simulink model "localDP_bs_env"  (R2020a)
settings: Solver=ode4  StartTime=0.0  StopTime=2000.0  FixedStep=1  RelTol=1e-3
InitFcn:
  | initial_data
values from neighbouring files (symbols this model uses):
  D1 = [MM1(1,1)/100, 0, 0; 0, MM1(2,2)/40, 0; 0, 0, MM1(3,3)/20]    [main.m]
  M1 = diag([6.25e5, 6.25e5, 6.25e5*7.5^2])    [main.m]
  Ma1 = [7.58e4, 0, 0; 0, 3.69e5 -1.4e5; 0, -1.4e5, 8.77e6]    [main.m]
undefined symbols (not defined in the file or in its folder): magnitude
libraries: simulink x2
settings Model: Creator=jiang  LastModifiedBy=jiang

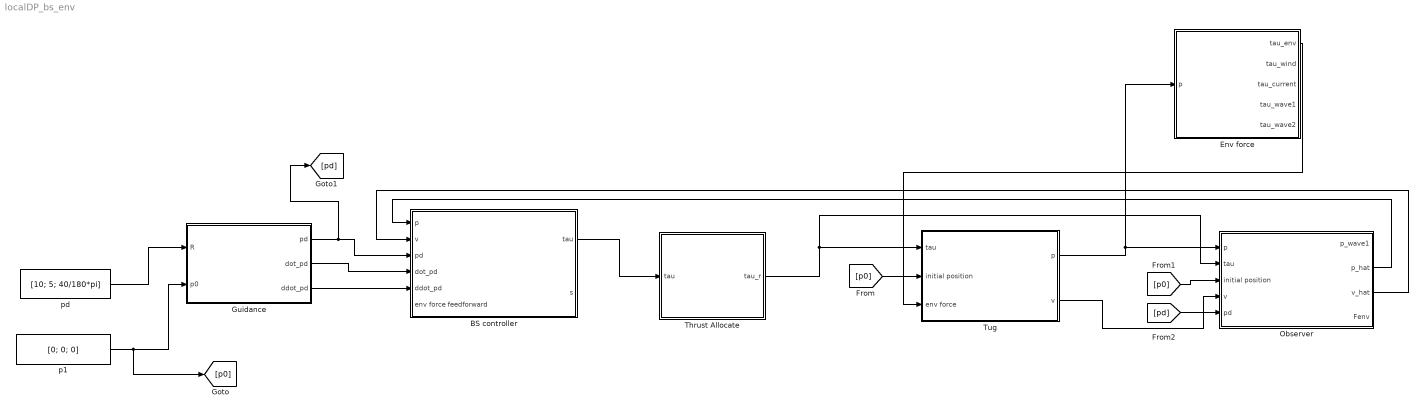
== system localDP_bs_env ==
  BS controller : Subsystem  mask{Kd=[2.5, 2.5, 2], Ki=[0.1, 0.1, 0.1], Gama=[0.7, 0.7, 0.7]}
      mask Display: disp("BS controller")
  Env force : Subsystem  mask{wind_speed=3, wind_angle=0, wind_ratio=0, current_speed=0.3, current_angle=0, current_ratio=0, wave_Hs=4.8, wave_Tp=13.4, wave_angle=0, wave1_ratio=1, wave2_ratio=1}
      mask prompts: wind_speed "wind speed"; wind_angle "wind angle"; wind_ratio "wind ratio"; current_speed "current speed"; current_angle "current angle"; current_ratio "current ratio"; wave_Hs "wave Hs"; wave_Tp "wave Tp"; wave_angle "wave angle"; wave1_ratio "wave1 ratio"; wave2_ratio "wave2 ratio"
      mask DialogControl ParameterGroupVar Prompt: wind parameters
      mask DialogControl Container5 Prompt: current parameters
      mask DialogControl wave Prompt: wave parameters
  Guidance : Subsystem  mask{T=[100, 100, 100]}
      mask prompts: T "时间常数"
  Observer : Subsystem  mask(wave spectrum damping ratio){lambda=[0.1 0.1 0.1], w_o=[0.469 0.469 0.469], K3=diag([1.4e4, 1.6e4, 2.5e6])*0.1, K4=diag([1.4e4, 1.6e4, 2.5e6]), w_c=0.6, T=diag([10 10 10])*100, Tp=13.4, wc_ratio=1.2}
      mask prompts: lambda "Relative damping ratio of wave spectrum: lambda"; w_o "Peak frequency of response spectrum: w_o (rad/s)"; K3 "Bias observer gain: K3"; K4 "Bias observer gain: K4"; w_c "Filter cut-off frequency: w_c (rad/s)"; T "Bias time constant: T (s)"; Tp "波浪谱峰周期"; wc_ratio "截至频率倍数（1.1~1.2）"
      mask init:
      | wo = [1, 1, 1] * 2 * pi / Tp;
      | wc = wo(1) * wc_ratio;
      | Zeta = 1;
      | Aw = blkdiag([0 1;-wo(1)^2 -2*lambda(1)*wo(1)],...
      |              [0 1;-wo(2)^2 -2*lambda(2)*wo(2)],...
      |              [0 1;-wo(3)^2 -2*lambda(3)*wo(3)]);
      | K1 = zeros(6,3);
      | for i =1:3
      |     K1(2*i-1,i) = -2*(Zeta - lambda(i))*wc/wo(i);
      |     K1(2*i,i) = 2*wo(i)*(Zeta - lambda(i));
      | end
      | K2 = diag([wc,wc,wc]);
      | Cw = zeros(3,6);
      | Cw(1,2) = 1;Cw(2,4) = 1;Cw(3,6) = 1;
      mask Display: disp('nonlinear passive observer')
  Thrust Allocate : Subsystem  mask{f0=[100;100;100], a0=[-50;60;-100]}
  Tug : Subsystem  mask{wv=on}
      mask prompts: wv "Display animation of the vessel's motion"
  p1 : Constant  Value=[0; 0; 0]
  pd : Constant  Value=[10; 5; 40/180*pi]
  wires:
  Thrust Allocate/1(tau_r) -> Observer/2(tau), Tug/1(tau)
  BS controller/1(tau) -> Thrust Allocate/1(tau)
  Env force/1(tau_env) -> Tug/3(env force)
  Tug/2(v) -> Observer/4(v)
  Tug/1(p) -> Env force/1(p), Observer/1(p)
  Observer/2(p_hat) -> BS controller/1(p)
  Observer/3(v_hat) -> BS controller/2(v)
  p1/1 -> [p0], Guidance/2(p0)
  pd/1 -> Guidance/1(R)
  Guidance/2(dot_pd) -> BS controller/4(dot_pd)
  Guidance/1(pd) -> [pd], BS controller/3(pd)
  Guidance/3(ddot_pd) -> BS controller/5(ddot_pd)
  [p0] -> Tug/2(initial position)
  [p0] -> Observer/3(initial position)
  [pd] -> Observer/5(pd)

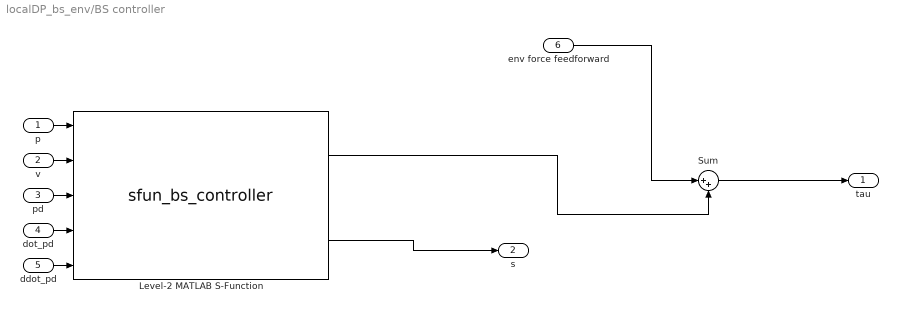
== system localDP_bs_env/BS controller ==
  p : Inport
  v : Inport  Port=2
  pd : Inport  Port=3
  dot_pd : Inport  Port=4
  ddot_pd : Inport  Port=5
  env force feedforward : Inport  Port=6
  Level-2 MATLAB S-Function : M-S-Function  FunctionName=sfun_bs_controller  Parameters=Kd, Ki, Gama
  Sum : Sum  Inputs=|++
  tau : Outport
  s : Outport  Port=2
  wires:
  Level-2 MATLAB S-Function/2 -> s/1
  v/1 -> Level-2 MATLAB S-Function/2
  p/1 -> Level-2 MATLAB S-Function/1
  pd/1 -> Level-2 MATLAB S-Function/3
  ddot_pd/1 -> Level-2 MATLAB S-Function/5
  dot_pd/1 -> Level-2 MATLAB S-Function/4
  Sum/1 -> tau/1
  Level-2 MATLAB S-Function/1 -> Sum/2
  env force feedforward/1 -> Sum/1

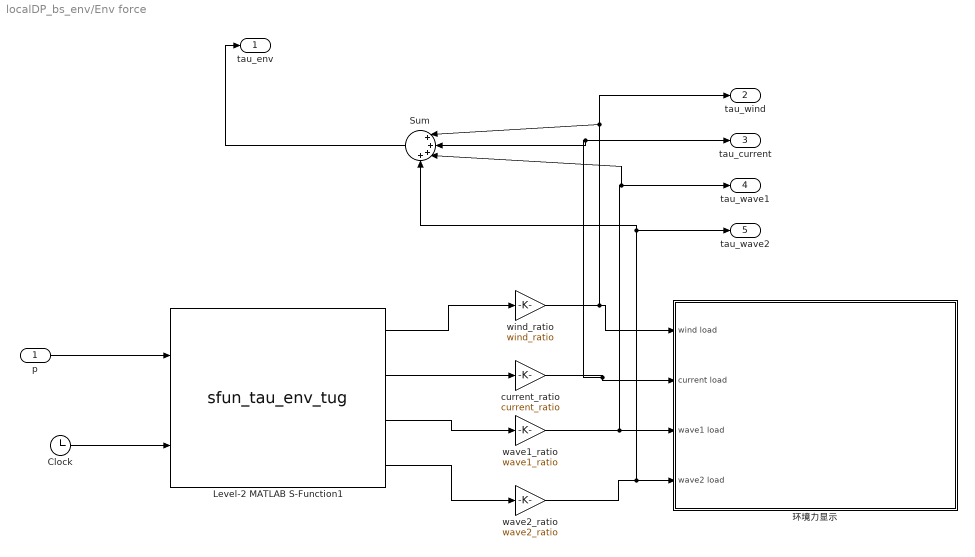
== system localDP_bs_env/Env force ==
  p : Inport
  Clock : Clock
  Level-2 MATLAB S-Function1 : M-S-Function  FunctionName=sfun_tau_env_tug  Parameters=wind_speed, wind_angle, current_speed, current_angle, wave_Hs, wave_Tp, wave_angle
  Sum : Sum  Inputs=|++++
  current_ratio : Gain  Gain=current_ratio
  wave1_ratio : Gain  Gain=wave1_ratio
  wave2_ratio : Gain  Gain=wave2_ratio
  wind_ratio : Gain  Gain=wind_ratio
  环境力显示 : Subsystem
  tau_env : Outport
  tau_wind : Outport  Port=2
  tau_current : Outport  Port=3
  tau_wave1 : Outport  Port=4
  tau_wave2 : Outport  Port=5
  wires:
  p/1 -> Level-2 MATLAB S-Function1/1
  Level-2 MATLAB S-Function1/1 -> wind_ratio/1
  Level-2 MATLAB S-Function1/2 -> current_ratio/1
  Level-2 MATLAB S-Function1/3 -> wave1_ratio/1
  Level-2 MATLAB S-Function1/4 -> wave2_ratio/1
  Clock/1 -> Level-2 MATLAB S-Function1/2
  wind_ratio/1 -> 环境力显示/1(wind load), tau_wind/1, Sum/1
  current_ratio/1 -> Sum/2, tau_current/1, 环境力显示/2(current load)
  wave1_ratio/1 -> Sum/3, tau_wave1/1, 环境力显示/3(wave1 load)
  wave2_ratio/1 -> Sum/4, tau_wave2/1, 环境力显示/4(wave2 load)
  Sum/1 -> tau_env/1

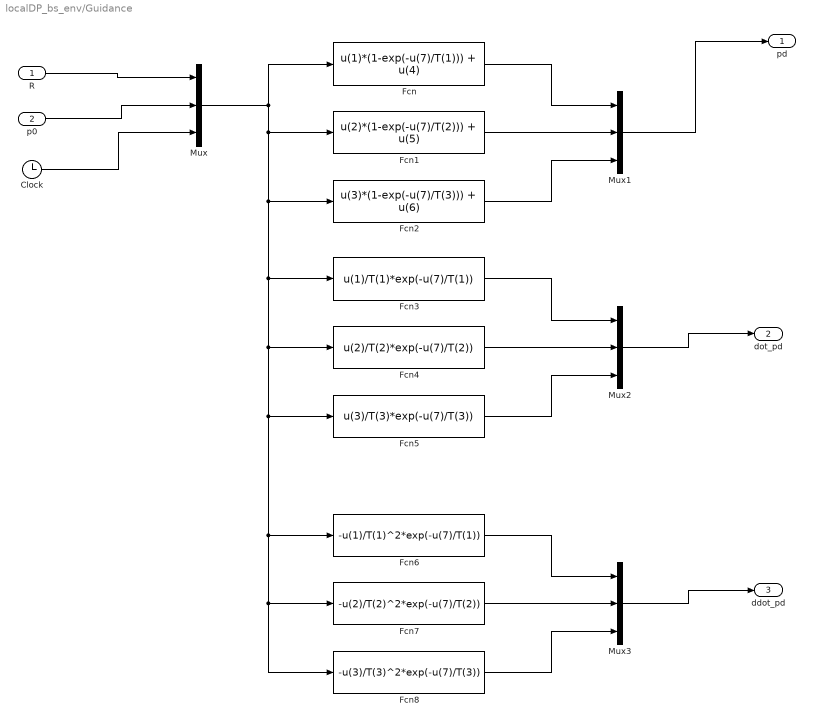
== system localDP_bs_env/Guidance ==
  R : Inport
  p0 : Inport  Port=2
  Clock : Clock
  Fcn : Fcn  Expr=u(1)*(1-exp(-u(7)/T(1))) + u(4)
  Fcn1 : Fcn  Expr=u(2)*(1-exp(-u(7)/T(2))) + u(5)
  Fcn2 : Fcn  Expr=u(3)*(1-exp(-u(7)/T(3))) + u(6)
  Fcn3 : Fcn  Expr=u(1)/T(1)*exp(-u(7)/T(1))
  Fcn4 : Fcn  Expr=u(2)/T(2)*exp(-u(7)/T(2))
  Fcn5 : Fcn  Expr=u(3)/T(3)*exp(-u(7)/T(3))
  Fcn6 : Fcn  Expr=-u(1)/T(1)^2*exp(-u(7)/T(1))
  Fcn7 : Fcn  Expr=-u(2)/T(2)^2*exp(-u(7)/T(2))
  Fcn8 : Fcn  Expr=-u(3)/T(3)^2*exp(-u(7)/T(3))
  Mux{,1..3} (4 alike) : Mux  Inputs=3
  pd : Outport
  dot_pd : Outport  Port=2
  ddot_pd : Outport  Port=3
  wires:
  Clock/1 -> Mux/3
  p0/1 -> Mux/2
  R/1 -> Mux/1
  Fcn/1 -> Mux1/1
  Fcn1/1 -> Mux1/2
  Fcn2/1 -> Mux1/3
  Mux1/1 -> pd/1
  Fcn5/1 -> Mux2/3
  Fcn4/1 -> Mux2/2
  Fcn3/1 -> Mux2/1
  Mux2/1 -> dot_pd/1
  Fcn7/1 -> Mux3/2
  Fcn6/1 -> Mux3/1
  Mux3/1 -> ddot_pd/1
  Mux/1 -> Fcn8/1, Fcn7/1, Fcn6/1, Fcn5/1, Fcn4/1, Fcn3/1, Fcn2/1, Fcn1/1, Fcn/1
  Fcn8/1 -> Mux3/3

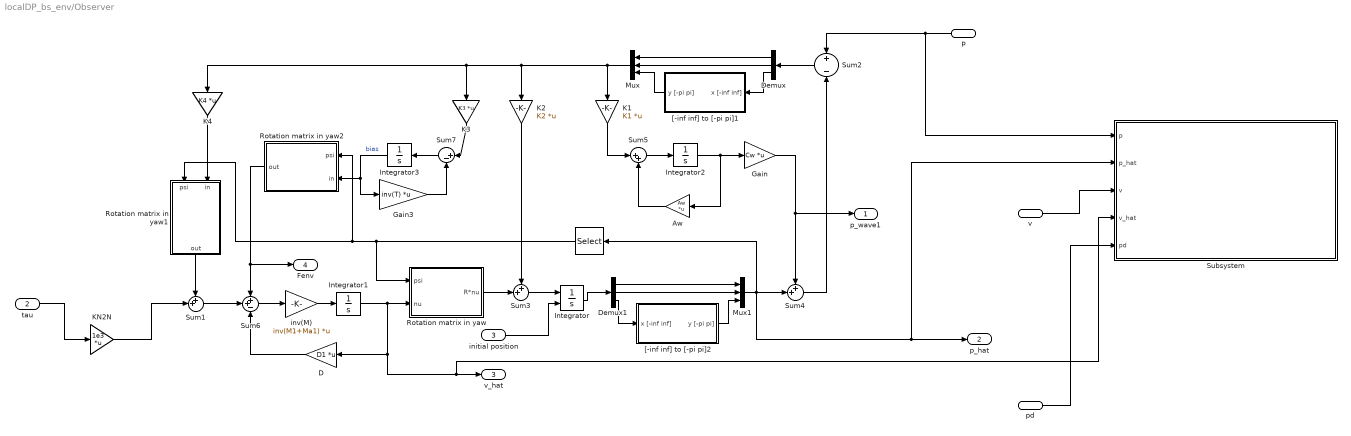
== system localDP_bs_env/Observer ==
  p : Inport
  tau : Inport  Port=2
  initial position : Inport  Port=3
  v : Inport  Port=4
  pd : Inport  Port=5
  " " : Selector  InputPortWidth=3  IndexOptions=Index vector (dialog)  Indices=[3]  OutputSizes=1
  Aw : Gain  Gain=Aw  Multiplication=Matrix(K*u)  SaturateOnIntegerOverflow=on  OutDataTypeStr=Inherit: Same as input  ParamDataTypeStr=Inherit: Same as input
  D : Gain  Gain=D1  Multiplication=Matrix(K*u)  SaturateOnIntegerOverflow=on  OutDataTypeStr=Inherit: Same as input  ParamDataTypeStr=Inherit: Same as input
  Demux : Demux  Outputs=3
  Demux1 : Demux  Outputs=3
  Gain : Gain  Gain=Cw  Multiplication=Matrix(K*u)
  Gain3 : Gain  Gain=inv(T)  Multiplication=Matrix(K*u)  SaturateOnIntegerOverflow=on  OutDataTypeStr=Inherit: Same as input  ParamDataTypeStr=Inherit: Same as input
  Integrator : Integrator  InitialConditionSource=external
  Integrator1 : Integrator
  Integrator2 : Integrator
  Integrator3 : Integrator
  K1 : Gain  Gain=K1  Multiplication=Matrix(K*u)  SaturateOnIntegerOverflow=on  OutDataTypeStr=Inherit: Same as input  ParamDataTypeStr=Inherit: Same as input
  K2 : Gain  Gain=K2  Multiplication=Matrix(K*u)  SaturateOnIntegerOverflow=on  OutDataTypeStr=Inherit: Same as input  ParamDataTypeStr=Inherit: Same as input
  K3 : Gain  Gain=K3  Multiplication=Matrix(K*u)  SaturateOnIntegerOverflow=on  OutDataTypeStr=Inherit: Same as input  ParamDataTypeStr=Inherit: Same as input
  K4 : Gain  Gain=K4  Multiplication=Matrix(K*u)  SaturateOnIntegerOverflow=on  OutDataTypeStr=Inherit: Same as input  ParamDataTypeStr=Inherit: Same as input
  KN2N : Gain  Gain=1e3  Multiplication=Matrix(K*u)  SaturateOnIntegerOverflow=on  OutDataTypeStr=Inherit: Same as input  ParamDataTypeStr=Inherit: Same as input
  Mux : Mux  Inputs=3
  Mux1 : Mux  Inputs=3
  Rotation matrix in yaw : Subsystem
  Rotation matrix in yaw1 : Subsystem
  Rotation matrix in yaw2 : Subsystem
  Subsystem : Subsystem
  Sum1 : Sum  Inputs=++|  InputSameDT=on  SaturateOnIntegerOverflow=on  OutDataTypeStr=Inherit: Same as first input
  Sum2 : Sum  Inputs=+|-  InputSameDT=on  SaturateOnIntegerOverflow=on  OutDataTypeStr=Inherit: Same as first input
  Sum3 : Sum  Inputs=++|  InputSameDT=on  SaturateOnIntegerOverflow=on  OutDataTypeStr=Inherit: Same as first input
  Sum4 : Sum  Inputs=++|  InputSameDT=on  SaturateOnIntegerOverflow=on  OutDataTypeStr=Inherit: Same as first input
  Sum5 : Sum  Inputs=|++  InputSameDT=on  SaturateOnIntegerOverflow=on  OutDataTypeStr=Inherit: Same as first input
  Sum6 : Sum  Inputs=++-  InputSameDT=on  SaturateOnIntegerOverflow=on  OutDataTypeStr=Inherit: Same as first input
  Sum7 : Sum  Inputs=|+-  InputSameDT=on  SaturateOnIntegerOverflow=on  OutDataTypeStr=Inherit: Same as first input
  "[-inf inf] to [-pi pi]1" : Subsystem  mask([-inf inf] to [-pi pi]){}
      mask help: Converts an angle in rad to (-pi pi)
  "[-inf inf] to [-pi pi]2" : Subsystem
  inv(M) : Gain  Gain=inv(M1+Ma1)  Multiplication=Matrix(K*u)  SaturateOnIntegerOverflow=on  OutDataTypeStr=Inherit: Same as input  ParamDataTypeStr=Inherit: Same as input
  p_wave1 : Outport
  p_hat : Outport  Port=2
  v_hat : Outport  Port=3
  Fenv : Outport  Port=4
  wires:
  tau/1 -> KN2N/1
  p/1 -> Subsystem/1(p), Sum2/1
  Gain3/1 -> Sum7/2
  Sum7/1 -> Integrator3/1
  Integrator3/1 -> Gain3/1, Rotation matrix in yaw2/2(in)  "bias"
  Sum4/1 -> Sum2/2
  Integrator/1 -> Demux1/1
  Sum3/1 -> Integrator/1
  Sum2/1 -> Demux/1
  Demux/3 -> "[-inf inf] to [-pi pi]1"/1(x [-inf inf])
  "[-inf inf] to [-pi pi]1"/1(y [-pi pi]) -> Mux/3
  Demux/1 -> Mux/1
  Demux/2 -> Mux/2
  Mux/1 -> K1/1, K2/1, K4/1, K3/1
  Demux1/1 -> Mux1/1
  Demux1/2 -> Mux1/2
  "[-inf inf] to [-pi pi]2"/1(y [-pi pi]) -> Mux1/3
  Demux1/3 -> "[-inf inf] to [-pi pi]2"/1(x [-inf inf])
  Mux1/1 -> Subsystem/2(p_hat), p_hat/1, Sum4/2, " "/1
  Sum5/1 -> Integrator2/1
  K1/1 -> Sum5/1
  Integrator2/1 -> Gain/1, Aw/1
  Aw/1 -> Sum5/2
  K2/1 -> Sum3/1
  Rotation matrix in yaw/1(R*nu) -> Sum3/2
  K3/1 -> Sum7/1
  inv(M)/1 -> Integrator1/1
  Sum6/1 -> inv(M)/1
  Integrator1/1 -> Rotation matrix in yaw/2(nu), D/1, Subsystem/4(v_hat), v_hat/1
  " "/1 -> Rotation matrix in yaw/1(psi), Rotation matrix in yaw1/1(psi), Rotation matrix in yaw2/1(psi)
  Sum1/1 -> Sum6/2
  D/1 -> Sum6/3
  K4/1 -> Rotation matrix in yaw1/2(in)
  Rotation matrix in yaw1/1(out) -> Sum1/1
  Rotation matrix in yaw2/1(out) -> Sum6/1, Fenv/1
  initial position/1 -> Integrator/2
  Gain/1 -> Sum4/1, p_wave1/1
  v/1 -> Subsystem/3(v)
  KN2N/1 -> Sum1/2
  pd/1 -> Subsystem/5(pd)

== system localDP_bs_env/Thrust Allocate ==
  tau : Inport
  Comparison between thrusts : Subsystem
  Level-2 MATLAB S-Function : M-S-Function  FunctionName=sfun_Thrust_Allocate  Parameters=f0, a0
  a : Scope
  f : Scope
  tau1 : Scope  NumInputPorts=3
  tau_r : Outport
  wires:
  tau/1 -> Comparison between thrusts/1(commanded thrust), Level-2 MATLAB S-Function/1
  Level-2 MATLAB S-Function/5 -> Comparison between thrusts/2(real thrust), tau_r/1
  Level-2 MATLAB S-Function/1 -> f/1
  Level-2 MATLAB S-Function/3 -> a/1
  Comparison between thrusts/1(surge direction) -> tau1/1
  Comparison between thrusts/2(sway direction) -> tau1/2
  Comparison between thrusts/3(yaw direction) -> tau1/3

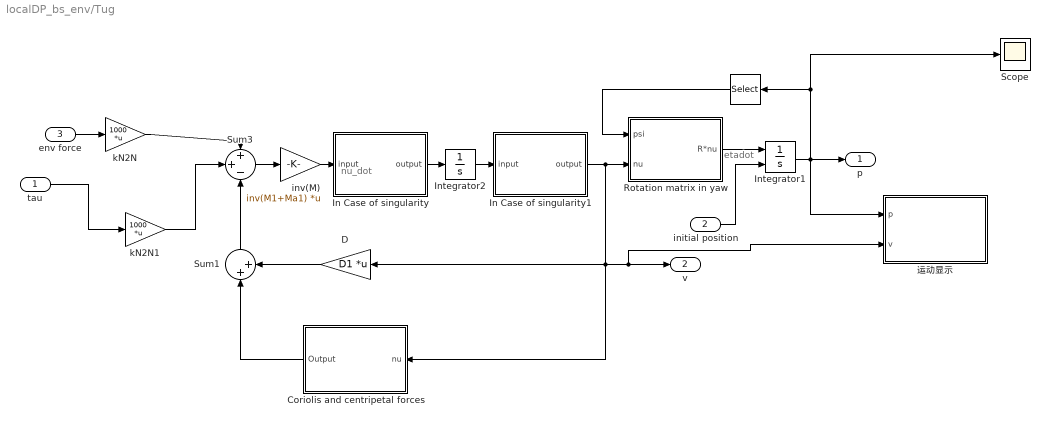
== system localDP_bs_env/Tug ==
  note: nu_dot
  note: etadot
  tau : Inport
  initial position : Inport  Port=2
  env force : Inport  Port=3
  " " : Selector  InputPortWidth=3  IndexOptions=Index vector (dialog)  Indices=[3]  OutputSizes=1
  Coriolis and centripetal forces : Subsystem
  D : Gain  Gain=D1  Multiplication=Matrix(K*u)  SaturateOnIntegerOverflow=on  OutDataTypeStr=Inherit: Same as input  ParamDataTypeStr=Inherit: Same as input
  In Case of singularity : Subsystem
  In Case of singularity1 : Subsystem
  Integrator1 : Integrator  InitialConditionSource=external  InitialCondition=1.05
  Integrator2 : Integrator
  Rotation matrix in yaw : Subsystem
  Scope : Scope
  Sum1 : Sum  Inputs=|++  InputSameDT=on  SaturateOnIntegerOverflow=on  OutDataTypeStr=Inherit: Same as first input
  Sum3 : Sum  Inputs=++-  InputSameDT=on  SaturateOnIntegerOverflow=on  OutDataTypeStr=Inherit: Same as first input
  inv(M) : Gain  Gain=inv(M1+Ma1)  Multiplication=Matrix(K*u)  SaturateOnIntegerOverflow=on  OutDataTypeStr=Inherit: Same as input  ParamDataTypeStr=Inherit: Same as input
  kN2N : Gain  Gain=1000  Multiplication=Matrix(K*u)  SaturateOnIntegerOverflow=on  OutDataTypeStr=Inherit: Same as input  ParamDataTypeStr=Inherit: Same as input
  kN2N1 : Gain  Gain=1000  Multiplication=Matrix(K*u)  SaturateOnIntegerOverflow=on  OutDataTypeStr=Inherit: Same as input  ParamDataTypeStr=Inherit: Same as input
  运动显示 : Subsystem
  p : Outport
  v : Outport  Port=2
  wires:
  Sum3/1 -> inv(M)/1
  inv(M)/1 -> In Case of singularity/1(input)
  Rotation matrix in yaw/1(R*nu) -> Integrator1/1
  Integrator1/1 -> 运动显示/1(p), p/1, Scope/1, " "/1
  " "/1 -> Rotation matrix in yaw/1(psi)
  tau/1 -> kN2N1/1
  initial position/1 -> Integrator1/2
  Sum1/1 -> Sum3/3
  env force/1 -> kN2N/1
  Integrator2/1 -> In Case of singularity1/1(input)
  In Case of singularity/1(output) -> Integrator2/1
  In Case of singularity1/1(output) -> Rotation matrix in yaw/2(nu), D/1, Coriolis and centripetal forces/1(nu), 运动显示/2(v), v/1
  D/1 -> Sum1/2
  Coriolis and centripetal forces/1(Output) -> Sum1/1
  kN2N/1 -> Sum3/1
  kN2N1/1 -> Sum3/2

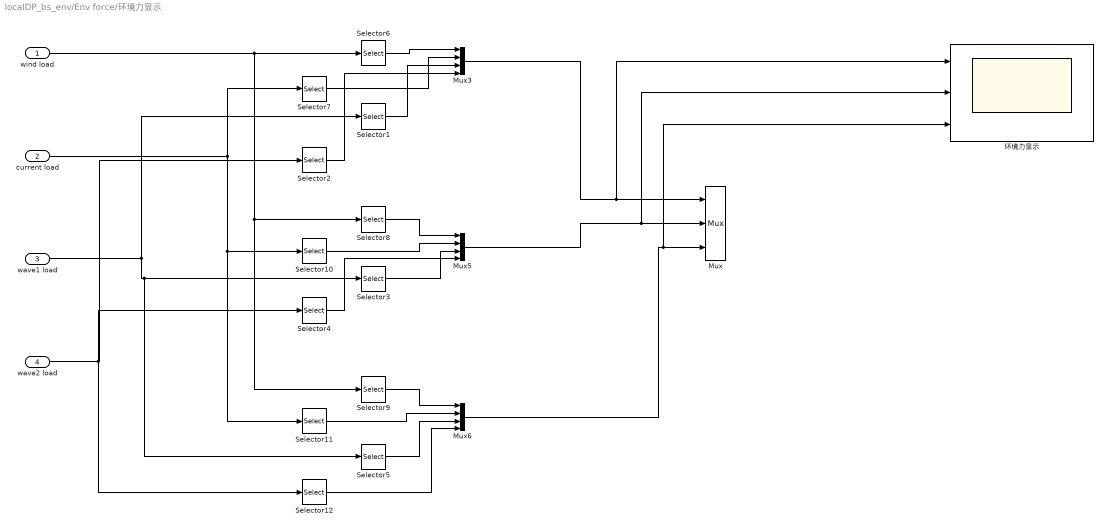
== system localDP_bs_env/Env force/环境力显示 ==
  wind load : Inport
  current load : Inport  Port=2
  wave1 load : Inport  Port=3
  wave2 load : Inport  Port=4
  Mux : Mux  Inputs=3
  Mux3 : Mux
  Mux5 : Mux
  Mux6 : Mux
  Selector{1..2,6..7} (4 alike) : Selector  InputPortWidth=3  IndexOptions=Index vector (dialog)  Indices=[1]  OutputSizes=1
  Selector{3..4,8,10} (4 alike) : Selector  InputPortWidth=3  IndexOptions=Index vector (dialog)  Indices=[2]  OutputSizes=1
  Selector{5,9,11..12} (4 alike) : Selector  InputPortWidth=3  IndexOptions=Index vector (dialog)  Indices=[3]  OutputSizes=1
  环境力显示 : Scope  NumInputPorts=3
  wires:
  Selector8/1 -> Mux5/1
  Mux3/1 -> 环境力显示/1, Mux/1
  Selector10/1 -> Mux5/2
  wind load/1 -> Selector9/1, Selector8/1, Selector6/1
  Selector7/1 -> Mux3/2
  Selector6/1 -> Mux3/1
  Selector9/1 -> Mux6/1
  Selector11/1 -> Mux6/2
  current load/1 -> Selector11/1, Selector10/1, Selector7/1
  Mux5/1 -> 环境力显示/2, Mux/2
  Mux6/1 -> 环境力显示/3, Mux/3
  wave1 load/1 -> Selector1/1, Selector5/1, Selector3/1
  Selector1/1 -> Mux3/3
  Selector2/1 -> Mux3/4
  Selector3/1 -> Mux5/3
  wave2 load/1 -> Selector12/1, Selector4/1, Selector2/1
  Selector4/1 -> Mux5/4
  Selector5/1 -> Mux6/3
  Selector12/1 -> Mux6/4

== system localDP_bs_env/Observer/Rotation matrix in yaw ==
  psi : Inport
  nu : Inport  Port=2
  Fcn : Fcn  Expr=cos(u(1))*u(2)-sin(u(1))*u(3)
  Fcn1 : Fcn  Expr=sin(u(1))*u(2)+cos(u(1))*u(3)
  Fcn2 : Fcn  Expr=u(4)
  Mux : Mux  Inputs=2
  Mux1 : Mux  Inputs=3
  R*nu : Outport
  wires:
  Mux1/1 -> R*nu/1  "eta_dot"
  Mux/1 -> Fcn/1, Fcn1/1, Fcn2/1
  psi/1 -> Mux/1
  nu/1 -> Mux/2
  Fcn1/1 -> Mux1/2  "y_dot"
  Fcn/1 -> Mux1/1  "x_dot"
  Fcn2/1 -> Mux1/3  "psi_dot"

== system localDP_bs_env/Observer/Rotation matrix in yaw1 ==
  psi : Inport
  in : Inport  Port=2
  Fcn : Fcn  Expr=cos(u(1))*u(2)+sin(u(1))*u(3)
  Fcn1 : Fcn  Expr=-sin(u(1))*u(2)+cos(u(1))*u(3)
  Fcn2 : Fcn  Expr=u(4)
  Mux : Mux  Inputs=2
  Mux1 : Mux  Inputs=3
  out : Outport
  wires:
  Fcn2/1 -> Mux1/3
  Fcn/1 -> Mux1/1
  Fcn1/1 -> Mux1/2
  in/1 -> Mux/2
  psi/1 -> Mux/1
  Mux/1 -> Fcn2/1, Fcn1/1, Fcn/1
  Mux1/1 -> out/1

== system localDP_bs_env/Observer/Rotation matrix in yaw2 ==
  psi : Inport
  in : Inport  Port=2
  Fcn : Fcn  Expr=cos(u(1))*u(2)+sin(u(1))*u(3)
  Fcn1 : Fcn  Expr=-sin(u(1))*u(2)+cos(u(1))*u(3)
  Fcn2 : Fcn  Expr=u(4)
  Mux : Mux  Inputs=2
  Mux1 : Mux  Inputs=3
  out : Outport
  wires:
  Mux1/1 -> out/1
  Mux/1 -> Fcn/1, Fcn1/1, Fcn2/1
  psi/1 -> Mux/1
  in/1 -> Mux/2
  Fcn1/1 -> Mux1/2
  Fcn/1 -> Mux1/1
  Fcn2/1 -> Mux1/3

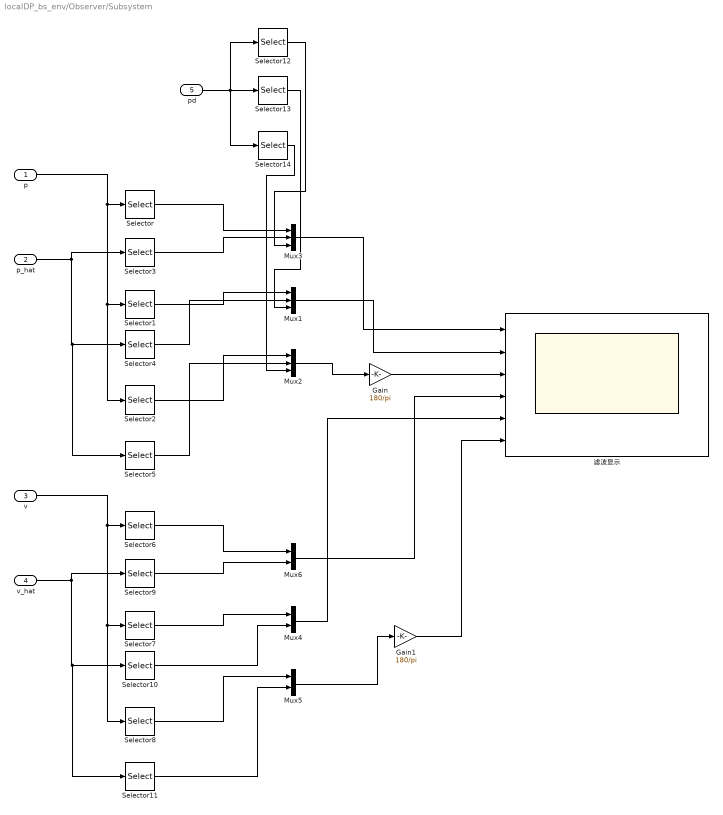
== system localDP_bs_env/Observer/Subsystem ==
  p : Inport
  p_hat : Inport  Port=2
  v : Inport  Port=3
  v_hat : Inport  Port=4
  pd : Inport  Port=5
  Gain : Gain  Gain=180/pi
  Gain1 : Gain  Gain=180/pi
  Mux1 : Mux  Inputs=3
  Mux2 : Mux  Inputs=3
  Mux3 : Mux  Inputs=3
  Mux4 : Mux  Inputs=2
  Mux5 : Mux  Inputs=2
  Mux6 : Mux  Inputs=2
  Selector{,3,6,9,12} (5 alike) : Selector  InputPortWidth=3  IndexOptions=Index vector (dialog)  Indices=[1 ]  OutputSizes=1
  Selector{1,4,7,10,13} (5 alike) : Selector  InputPortWidth=3  IndexOptions=Index vector (dialog)  Indices=[2 ]  OutputSizes=1
  Selector{2,5,8,11,14} (5 alike) : Selector  InputPortWidth=3  IndexOptions=Index vector (dialog)  Indices=[3 ]  OutputSizes=1
  滤波显示 : Scope  NumInputPorts=6
  wires:
  p/1 -> Selector2/1, Selector1/1, Selector/1
  Selector/1 -> Mux3/1
  p_hat/1 -> Selector5/1, Selector4/1, Selector3/1
  Selector3/1 -> Mux3/2
  Mux3/1 -> 滤波显示/1
  Mux1/1 -> 滤波显示/2
  Mux2/1 -> Gain/1
  Mux5/1 -> Gain1/1
  v/1 -> Selector8/1, Selector7/1, Selector6/1
  v_hat/1 -> Selector11/1, Selector10/1, Selector9/1
  Mux6/1 -> 滤波显示/4
  Mux4/1 -> 滤波显示/5
  Selector1/1 -> Mux1/1
  Selector4/1 -> Mux1/2
  Selector2/1 -> Mux2/1
  Selector5/1 -> Mux2/2
  Selector6/1 -> Mux6/1
  Selector9/1 -> Mux6/2
  Selector7/1 -> Mux4/1
  Selector10/1 -> Mux4/2
  Selector8/1 -> Mux5/1
  Selector11/1 -> Mux5/2
  Gain/1 -> 滤波显示/3
  Gain1/1 -> 滤波显示/6
  pd/1 -> Selector14/1, Selector13/1, Selector12/1
  Selector12/1 -> Mux3/3
  Selector13/1 -> Mux1/3
  Selector14/1 -> Mux2/3

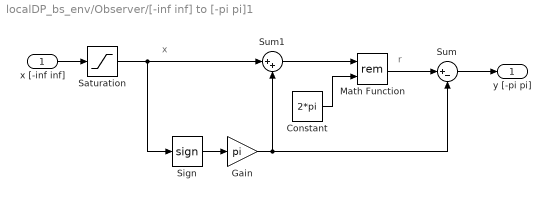
== system localDP_bs_env/Observer/[-inf inf] to [-pi pi]1 ==
  note: x
  note: r
  x [-inf inf] : Inport
  Constant : Constant  Value=2*pi
  Gain : Gain  Gain=pi  SaturateOnIntegerOverflow=on  OutDataTypeStr=Inherit: Same as input  ParamDataTypeStr=Inherit: Same as input
  Math Function : Math  Operator=rem  SignedPower=on  SaturateOnIntegerOverflow=on
  Saturation : Saturate  UpperLimit=1e10  LowerLimit=-1e10
  Sign : Signum
  Sum : Sum  Inputs=|+-  SaturateOnIntegerOverflow=on
  Sum1 : Sum  Inputs=|++  SaturateOnIntegerOverflow=on
  y [-pi pi] : Outport
  wires:
  x [-inf inf]/1 -> Saturation/1
  Sign/1 -> Gain/1
  Gain/1 -> Sum/2, Sum1/2
  Sum1/1 -> Math Function/1
  Constant/1 -> Math Function/2
  Math Function/1 -> Sum/1
  Sum/1 -> y [-pi pi]/1
  Saturation/1 -> Sum1/1, Sign/1

== system localDP_bs_env/Observer/[-inf inf] to [-pi pi]2 ==
  note: r
  note: x
  x [-inf inf] : Inport
  Constant : Constant  Value=2*pi
  Gain : Gain  Gain=pi  SaturateOnIntegerOverflow=on  OutDataTypeStr=Inherit: Same as input  ParamDataTypeStr=Inherit: Same as input
  Math Function : Math  Operator=rem  SignedPower=on  SaturateOnIntegerOverflow=on
  Saturation : Saturate  UpperLimit=1e10  LowerLimit=-1e10
  Sign : Signum
  Sum : Sum  Inputs=|+-  SaturateOnIntegerOverflow=on
  Sum1 : Sum  Inputs=|++  SaturateOnIntegerOverflow=on
  y [-pi pi] : Outport
  wires:
  Saturation/1 -> Sign/1, Sum1/1
  Sum/1 -> y [-pi pi]/1
  Math Function/1 -> Sum/1
  Constant/1 -> Math Function/2
  Sum1/1 -> Math Function/1
  Gain/1 -> Sum1/2, Sum/2
  Sign/1 -> Gain/1
  x [-inf inf]/1 -> Saturation/1

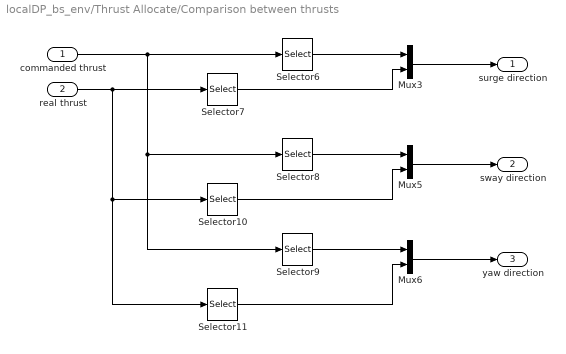
== system localDP_bs_env/Thrust Allocate/Comparison between thrusts ==
  commanded thrust : Inport
  real thrust : Inport  Port=2
  Mux3 : Mux  Inputs=2
  Mux5 : Mux  Inputs=2
  Mux6 : Mux  Inputs=2
  Selector10 : Selector  InputPortWidth=3  IndexOptions=Index vector (dialog)  Indices=[2]  OutputSizes=1
  Selector11 : Selector  InputPortWidth=3  IndexOptions=Index vector (dialog)  Indices=[3]  OutputSizes=1
  Selector6 : Selector  InputPortWidth=3  IndexOptions=Index vector (dialog)  Indices=[1]  OutputSizes=1
  Selector7 : Selector  InputPortWidth=3  IndexOptions=Index vector (dialog)  Indices=[1]  OutputSizes=1
  Selector8 : Selector  InputPortWidth=3  IndexOptions=Index vector (dialog)  Indices=[2]  OutputSizes=1
  Selector9 : Selector  InputPortWidth=3  IndexOptions=Index vector (dialog)  Indices=[3]  OutputSizes=1
  surge direction : Outport
  sway direction : Outport  Port=2
  yaw direction : Outport  Port=3
  wires:
  Selector9/1 -> Mux6/1
  Selector11/1 -> Mux6/2
  Selector10/1 -> Mux5/2
  Selector8/1 -> Mux5/1
  Selector7/1 -> Mux3/2
  Selector6/1 -> Mux3/1
  Mux3/1 -> surge direction/1
  Mux5/1 -> sway direction/1
  Mux6/1 -> yaw direction/1
  commanded thrust/1 -> Selector6/1, Selector8/1, Selector9/1
  real thrust/1 -> Selector7/1, Selector10/1, Selector11/1

== system localDP_bs_env/Tug/Coriolis and centripetal forces ==
  nu : Inport
  Mux : Mux  Inputs=3
  Selector1 : Selector  InputPortWidth=3  IndexOptions=Index vector (dialog)  Indices=[1 ]  OutputSizes=1
  Selector2 : Selector  InputPortWidth=3  IndexOptions=Index vector (dialog)  Indices=[2]  OutputSizes=1
  Selector3 : Selector  InputPortWidth=3  IndexOptions=Index vector (dialog)  Indices=[3]  OutputSizes=1
  Subsystem : Subsystem
  Subsystem1 : Subsystem
  Subsystem2 : Subsystem
  Output : Outport
  wires:
  nu/1 -> Selector1/1, Selector2/1, Selector3/1
  Selector2/1 -> Subsystem/1(v), Subsystem2/2(v)  "v"
  Selector3/1 -> Subsystem/2(r), Subsystem1/2(r), Subsystem2/3(r)  "r"
  Selector1/1 -> Subsystem1/1(u), Subsystem2/1(u)  "u"
  Subsystem/1(x direction) -> Mux/1
  Subsystem1/1(y direction) -> Mux/2
  Subsystem2/1(yaw direction) -> Mux/3
  Mux/1 -> Output/1

== system localDP_bs_env/Tug/In Case of singularity ==
  input : Inport
  Compare To Constant : simulink/Logic and Bit Operations/Compare To Constant  relop=>=  const=1e8  OutDataTypeStr=boolean
  Stop Simulation : Stop
  output : Outport
  wires:
  input/1 -> output/1, Compare To Constant/1
  Compare To Constant/1 -> Stop Simulation/1

== system localDP_bs_env/Tug/In Case of singularity1 ==
  input : Inport
  Compare To Constant : simulink/Logic and Bit Operations/Compare To Constant  relop=>=  const=1e10  OutDataTypeStr=boolean
  Stop Simulation : Stop
  output : Outport
  wires:
  input/1 -> output/1, Compare To Constant/1
  Compare To Constant/1 -> Stop Simulation/1

== system localDP_bs_env/Tug/Rotation matrix in yaw ==
  psi : Inport
  nu : Inport  Port=2
  Fcn : Fcn  Expr=cos(u(1))*u(2)-sin(u(1))*u(3)
  Fcn1 : Fcn  Expr=sin(u(1))*u(2)+cos(u(1))*u(3)
  Fcn2 : Fcn  Expr=u(4)
  Mux : Mux  Inputs=2
  Mux1 : Mux  Inputs=3
  R*nu : Outport
  wires:
  Mux1/1 -> R*nu/1  "eta_dot"
  Mux/1 -> Fcn/1, Fcn1/1, Fcn2/1
  psi/1 -> Mux/1
  nu/1 -> Mux/2
  Fcn1/1 -> Mux1/2  "y_dot"
  Fcn/1 -> Mux1/1  "x_dot"
  Fcn2/1 -> Mux1/3  "psi_dot"

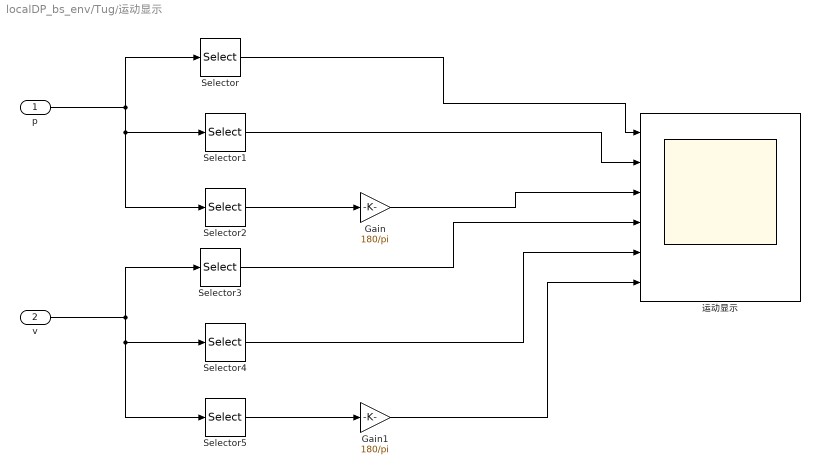
== system localDP_bs_env/Tug/运动显示 ==
  p : Inport
  v : Inport  Port=2
  Gain : Gain  Gain=180/pi
  Gain1 : Gain  Gain=180/pi
  Selector : Selector  InputPortWidth=3  IndexOptions=Index vector (dialog)  Indices=[1]  OutputSizes=1
  Selector1 : Selector  InputPortWidth=3  IndexOptions=Index vector (dialog)  Indices=[2]  OutputSizes=1
  Selector2 : Selector  InputPortWidth=3  IndexOptions=Index vector (dialog)  Indices=[3]  OutputSizes=1
  Selector3 : Selector  InputPortWidth=3  IndexOptions=Index vector (dialog)  Indices=[1]  OutputSizes=1
  Selector4 : Selector  InputPortWidth=3  IndexOptions=Index vector (dialog)  Indices=[2]  OutputSizes=1
  Selector5 : Selector  InputPortWidth=3  IndexOptions=Index vector (dialog)  Indices=[3]  OutputSizes=1
  运动显示 : Scope  NumInputPorts=6
  wires:
  p/1 -> Selector/1, Selector2/1, Selector1/1
  Selector2/1 -> Gain/1
  Selector/1 -> 运动显示/1
  Selector1/1 -> 运动显示/2
  Gain/1 -> 运动显示/3
  Selector4/1 -> 运动显示/5
  Gain1/1 -> 运动显示/6
  Selector5/1 -> Gain1/1
  Selector3/1 -> 运动显示/4
  v/1 -> Selector3/1, Selector5/1, Selector4/1

== system localDP_bs_env/Tug/Coriolis and centripetal forces/Subsystem ==
  v : Inport
  r : Inport  Port=2
  -a22 : Gain  Gain=-M1(2,2)-Ma1(2,2)  Multiplication=Matrix(K*u)  SaturateOnIntegerOverflow=on  OutDataTypeStr=Inherit: Same as input  ParamDataTypeStr=Inherit: Same as input
  -a26 : Gain  Gain=-M1(2,3)-Ma1(2,3)  Multiplication=Matrix(K*u)  SaturateOnIntegerOverflow=on  OutDataTypeStr=Inherit: Same as input  ParamDataTypeStr=Inherit: Same as input
  Add : Sum
  Math Function : Math  Operator=magnitude^2  SignedPower=on  SaturateOnIntegerOverflow=on
  Product : Product  RndMeth=Zero
  x direction : Outport
  wires:
  v/1 -> Product/1
  r/1 -> Product/2, Math Function/1
  Product/1 -> -a22/1
  Math Function/1 -> -a26/1
  -a22/1 -> Add/1
  -a26/1 -> Add/2
  Add/1 -> x direction/1

== system localDP_bs_env/Tug/Coriolis and centripetal forces/Subsystem1 ==
  u : Inport
  r : Inport  Port=2
  Product : Product  RndMeth=Zero
  a11 : Gain  Gain=M1(1,1)+Ma1(1,1)  Multiplication=Matrix(K*u)  SaturateOnIntegerOverflow=on  OutDataTypeStr=Inherit: Same as input  ParamDataTypeStr=Inherit: Same as input
  y direction : Outport
  wires:
  Product/1 -> a11/1
  r/1 -> Product/2
  u/1 -> Product/1
  a11/1 -> y direction/1

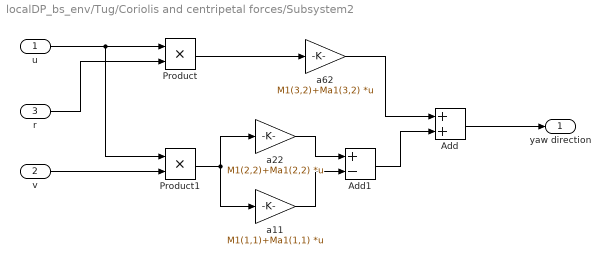
== system localDP_bs_env/Tug/Coriolis and centripetal forces/Subsystem2 ==
  u : Inport
  v : Inport  Port=2
  r : Inport  Port=3
  Add : Sum
  Add1 : Sum  Inputs=+-
  Product : Product  RndMeth=Zero
  Product1 : Product  RndMeth=Zero
  a11 : Gain  Gain=M1(1,1)+Ma1(1,1)  Multiplication=Matrix(K*u)  SaturateOnIntegerOverflow=on  OutDataTypeStr=Inherit: Same as input  ParamDataTypeStr=Inherit: Same as input
  a22 : Gain  Gain=M1(2,2)+Ma1(2,2)  Multiplication=Matrix(K*u)  SaturateOnIntegerOverflow=on  OutDataTypeStr=Inherit: Same as input  ParamDataTypeStr=Inherit: Same as input
  a62 : Gain  Gain=M1(3,2)+Ma1(3,2)  Multiplication=Matrix(K*u)  SaturateOnIntegerOverflow=on  OutDataTypeStr=Inherit: Same as input  ParamDataTypeStr=Inherit: Same as input
  yaw direction : Outport
  wires:
  u/1 -> Product/1, Product1/1
  r/1 -> Product/2
  Product/1 -> a62/1
  v/1 -> Product1/2
  Product1/1 -> a22/1, a11/1
  a22/1 -> Add1/1
  a11/1 -> Add1/2
  Add1/1 -> Add/2
  a62/1 -> Add/1
  Add/1 -> yaw direction/1
